simulink model "ContinousQP_Problem"  (R2021a)
settings: Solver=ode4  StartTime=0.0  StopTime=0.1  FixedStep=0.1  RelTol=1e-3
settings Model: Creator=isak.skeie  LastModifiedBy=isak.skeie

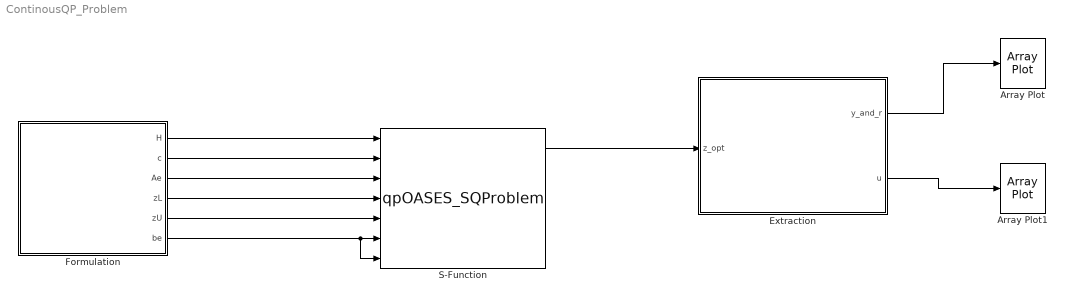
== system ContinousQP_Problem ==
  Array Plot : ArrayPlot  WindowPosition=[1.000000,41.000000,2560.000000,1377.000000,]  PlotType=Line  YLimits=[-0.23461784308342784,1.1605836801644394]  ShowLegend=on  DefaultConfigurationName=dsp.scopes.ArrayPlotBlockSpecification
  Array Plot1 : ArrayPlot  WindowPosition=[1.000000,41.000000,2560.000000,1377.000000,]  PlotType=Line  YLimits=[-6.0093032518257985,6.01137489480307]  ShowLegend=on  DefaultConfigurationName=dsp.scopes.ArrayPlotBlockSpecification
  Extraction : MATLAB Function  TreatAsAtomicUnit=on
  Formulation : MATLAB Function  TreatAsAtomicUnit=on
  S-Function : S-Function  FunctionName=qpOASES_SQProblem  SFunctionDeploymentMode=off  EnableBusSupport=off
  wires:
  Formulation/1(H) -> S-Function/1
  Formulation/2(c) -> S-Function/2
  Formulation/3(Ae) -> S-Function/3
  Formulation/4(zL) -> S-Function/4
  Formulation/5(zU) -> S-Function/5
  Formulation/6(be) -> S-Function/7, S-Function/6
  S-Function/1 -> Extraction/1(z_opt)
  Extraction/2(u) -> Array Plot1/1
  Extraction/1(y_and_r) -> Array Plot/1

== matlab function ContinousQP_Problem/Extraction ==
  data: z_opt input; y_and_r output; u output
function [y_and_r,u] = extract_results(z_opt) 

    N = 120; %prediction horizon length
    nx = 4; nu = 1; ny = 2; %no. of states, inputs and outputs
    
    %extract results
    Ua = z_opt(1+N*(0) :N*(nu),1); %control inputs
    Xa = z_opt(1+N*(nu) :N*(nu+nx),:); %states
    Ea = z_opt(1+N*(nu+nx) :N*(nu+nx+ny),:); %error in tracking
    Ya = z_opt(1+N*(nu+nx+ny) :N*(nu+nx+ny+ny),:); %outputs
    %we use the reshape function to rearrange the data
    y_temp = reshape(Ya,ny,N);%arranged outputs(rows as signals, columns as data)
    %the array plot in Simulink accepts signals in a format such that the columns 
    %represent the different signals and the rows represent the data for each  signal. So we need to transpose it.
    %The first column is for output y1 (angle), second column for output y2
    %(cart postion)
    y = y_temp';
    %Let us also plot the reference signals along with the output signals for
    %better viewing. 
    r = [zeros(N,1),[zeros(N/2,1);ones(N/2,1)]];
    
    %Put it as the third column (for r1) and fourth column (for r2).
    y_and_r = [y,r(:,1),r(:,2)];
    u_temp = reshape(Ua,nu,N); %arranged input(row as signals, columns as data)
    u = u_temp';

== matlab function ContinousQP_Problem/Formulation ==
  data: H output; c output; Ae output; zL output; zU output; be output
function [H,c,Ae,zL,zU,be] = QP_formulation_IVP()
%discrete time model
A = [1.0745,0.1025,0,0;
     1.5079,1.0745,0,0;
     -0.0248,-0.0008,1,0.1;
     -0.5026, -0.0248,0,1];
 
B = [-0.0025;-0.0512;0.0025;0.0504];
C = [1,0,0,0;0,0,1,0];
N = 120; % prediction horizon length

% set up the references for the whole prediction horizon length
r = [zeros(1,N); % first row for first output (pendulum angle)
 zeros(1,N/2) ones(1,N/2)]; % second row for second output (cart position)

%initial values of the states should be known or estimated
x0 = [0; 0; 0; 0];
%size of matrices
nx = 4; ny = 2; nu = 1;

%size of the unknow vector z
nz = N*(nx + nu + 2*ny);

%weighting matrices
Q=diag([1.0 1.0]); %tuning weight for error: there are 2
P=1e-3; %tuning weight for inputs: there is 1

% build matrices
H11 = kron(eye(N),P);
H22 = zeros(N*nx,N*nx);
H33 = kron(eye(N),Q);
H44 = zeros(N*ny,N*ny);
H_mat = blkdiag(H11,H22,H33,H44);

%qpOASES does not accept matrices, but only vectors
%we have to change H matrix to vector by stacking elements column wise
H = H_mat(:);
c = zeros(nz,1);

%constraints (from process model)
% from eq 3.33: state equation
Ae1u = -kron(eye(N),B);
Ae1x = eye(N*nx)-kron(diag(ones(N-abs(-1),1),-1),A);
Ae1e = zeros(N*nx,N*ny); 
Ae1y = zeros(N*nx,N*ny);
be1 = [A*x0;zeros((N-1)*nx,1)];

%from eq 3.34: measurement equation
Ae2u = zeros(N*ny,N*nu); 
Ae2x = -kron(eye(N),C);
Ae2e = zeros(N*ny,N*ny);
Ae2y = eye(N*ny);
be2 = zeros(N*ny,1);

%from eq 3.35: error equation
Ae3u = zeros(N*ny,N*nu); 
Ae3x = zeros(N*ny,N*nx);
Ae3e = eye(N*ny);
Ae3y = eye(N*ny);

% since be3 contains the reference vector in specific order, we have to use
% the function “reshape” to put the reference values in the right order
be3 = reshape(r,N*ny,1);
Ae_mat=[Ae1u Ae1x Ae1e Ae1y;
 Ae2u Ae2x Ae2e Ae2y;
 Ae3u Ae3x Ae3e Ae3y];

%qpOASES does not accept matrices, but only vectors
%we have to change Ae matrix to vector by stacking elements column wise 
Ae = Ae_mat(:); %stacking column wise
% make the standard be vector
be=[be1;be2;be3];

%bounds (not specified so assume between –inf to +inf)
zL=(-Inf*ones(nz,1));
zU=(Inf*ones(nz,1));
H_mat = blkdiag(H11,H22,H33,H44);

%qpOASES does not accept matrices, but only vectors
%we have to change H matrix to vector by stacking elements column wise
H = H_mat(:);
Ae_mat=[Ae1u Ae1x Ae1e Ae1y;
 Ae2u Ae2x Ae2e Ae2y;
 Ae3u Ae3x Ae3e Ae3y];

%qpOASES does not accept matrices, but only vectors
%we have to change Ae matrix to vector by stacking elements column wise 
Ae = Ae_mat(:); %stacking column wise
